simulink model "RobotSim"  (R2024b)
settings: Solver=ode45  StartTime=0.0  StopTime=100  MaxStep=0.1  RelTol=1e-3  EnableMultiTasking=on
InitFcn:
  | % LRS TU KL %
  | % By Alen Turnwald %
  | % 09.01.2017 %
  | clc
  | close
  | 
  | %% g_q
  | g_q = [1;0];
  | 
  | 
  | if ~exist('mp','var')||~exist('mc','var')||~exist('L','var')||~exist('g','var')||~exist('d1','var')||~exist('d2','var')
  | % Model Paramter
  |     warning(['(Some) Model Parameter are not defined!' ,10, '****  Setting the predefined parameter  ****'])
  |     N = 2;
  |     mc = 1.5;
  |     mp = 0.5;
  |     g = 9.82;
  |     L = 1;
  | % Damping factors
  |     d1 = 1e-2;
  |     d2 = 1e-2;
  | end
  | 
  | if ~exist('x_0','var')
  | % Initial state
  |     warning(['(Initial state "x_0" not defined or wrongly named!' ,10, '****  Setting x_0 = [0.1; 10 deg; 0; 0]  ****'])
  |     x_0 = zeros(4,1);
  |     x_0(1) = 0.1;
  |     x_0(2) = 10*pi/180;
  | end
  | 
  | if ~exist('K_lqr','var')||~exist('Kd_lqr','var')
  |     warning(['(No controller found!' ,10, '****   Applying a predefined controller  ****'])
  |     K_lqr = [-14.1421  171.8846  -25.2787   54.7535];
  | end
StopFcn:
  | %% load data
  | 
  | load output
  | 
  | %% Read data
  | q1 = out.Data(:,1);
  | q2 = out.Data(:,2)*180/pi;
  | x_ref = out.Data(:,5);
  | t = out.Time;
  | 
  | 
  | %% Plot
  | % close all
  | figure(2)
  | clf
  | h(1) = subplot(2,1,1);
  | plot(t,q1,'b','LineWidth',2); grid on
  | 
  | hold on
  | plot(t,x_ref,'r--')
  | hold off
  | ylabel('q_1 [m]')
  | legend('q_1','q_1 ref')
  | 
  | h(2) = subplot(2,1,2);
  | plot(t,q2,'b','LineWidth',2); grid on
  | hold on
  | plot(t,zeros(1,length(t)),'r--')
  | hold off
  | ylabel('q_2 [°]')
  | legend('q_2','q_2 ref')
  | 
  | xlabel('t [s]')
  | 
  | linkaxes(h,'x')
values from neighbouring files (symbols this model uses):
  l = 0.08    [robot.m]    (also in robot_cascade.m; robot_linear.m)
  m = 0.33    [robot.m]    (also in robot_cascade.m; robot_linear.m; robot_lqr.m)
  M = 1.180    (= 1.18)    [robot.m]    (also in robot_cascade.m; robot_linear.m; robot_lqr.m)
settings Model: Creator=Turnwald  LastModifiedBy=cosr3
settings SolverCC: AlgebraicLoopSolver=TrustRegion
settings DataIOCC: SaveFormat=Array  ReturnWorkspaceOutputs=off
settings OptimizationCC: OptimizeBlockIOStorage=off  BufferReuse=off  GlobalBufferReuse=off  ExpressionFolding=off  LocalBlockOutputs=off  LifeSpan=inf
settings DebuggingCC: SolverPrmCheckMsg=warning  UnconnectedInputMsg=warning  UnconnectedOutputMsg=warning  UnconnectedLineMsg=warning  AllowSymbolicDim=off  SFUnexpectedBacktrackingDiag=warning  SFNoUnconditionalDefaultTransitionDiag=warning  SFExecutionAtInitializationDiag=none  ArithmeticOperatorsInVariantConditions=warning
settings HardwareCC: ProdBitPerPointer=32  ProdBitPerSizeT=32  ProdBitPerPtrDiffT=32  ProdLargestAtomicFloat=None  ProdIntDivRoundTo=Undefined  ProdEndianess=Unspecified  ProdWordSize=32  ProdHWDeviceType=32-bit Generic
settings ModelReferenceCC: EnableRefExpFcnMdlSchedulingChecks=on  PropagateSignalLabelsOutOfModel=off
settings SFSimCC: SimUseLocalCustomCode=off  CustomCodeUndefinedFunction=UseInterfaceOnly
settings RTWCC: RTWUseLocalCustomCode=off  GPUComputeCapability=3.5
settings CodeAppCC: StateflowObjectComments=on
settings GRTTargetCC: TargetLangStandard=C89/C90 (ANSI)
settings ConfigComp: CovMetricSettings=dw  CovSaveCumulativeToWorkspaceVar=on  CovSaveSingleToWorkspaceVar=on  CovExternalEMLEnable=off

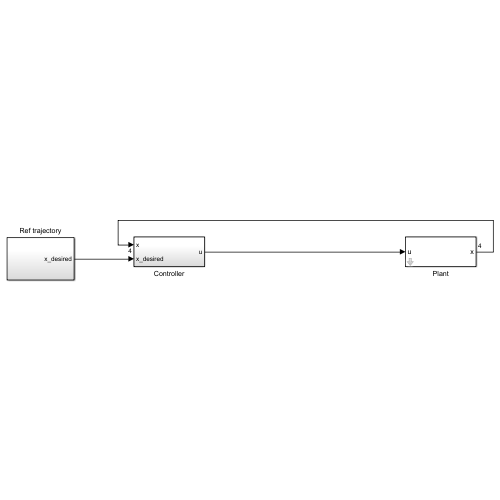
[thumbnail: Simulink's stored preview of the top-level diagram]
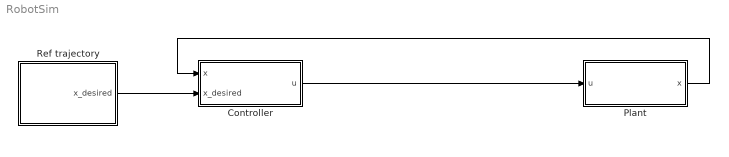
== system RobotSim ==
  Controller : Subsystem
  Plant : Subsystem  mask{mp=m, mc=M, L=l, g=g, g_q=g_q, d1=d1, d2=d2, x_0=x_0}
      mask help:
      | ---------------------------
      | TU Kaiserslautern, LRS
      | Ali Turnwald
      | Last Edit: 19.11.2015
      | ---------------------------
      |
      |
      | A non-linear model for the cart-pendulum system for simulation and animation
      |
      | mc = Mass of the cart
      | mp = Mass of the pendulum
      | g =  Earth gravity
      | L =  Length of the pendulum
      | d1 = Damping of the cart displacement
      | d2 = Damping in the joint
      | x_0 = The vector af initail state [4x1]
      mask DialogControl Text Prompt: Cart-Pendulum System
      mask Display:
      | port_label('output', 1, 'x')
      | port_label('input', 1, 'u')
  Ref trajectory : Subsystem
  wires:
  Ref trajectory/1(x_desired) -> Controller/2(x_desired)
  Plant/1(x) -> Controller/1(x)
  Controller/1(u) -> Plant/1(u)

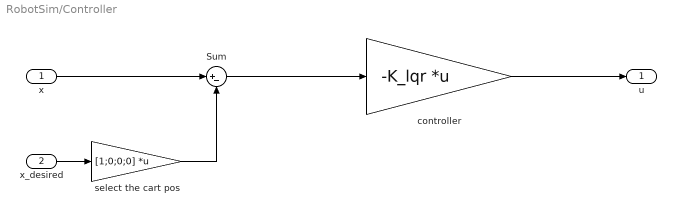
== system RobotSim/Controller ==
  x : Inport
  x_desired : Inport  Port=2
  Sum : Sum  Inputs=|+-
  controller : Gain  Gain=-K_lqr  Multiplication=Matrix(K*u)
  select the cart pos : Gain  Gain=[1;0;0;0]  Multiplication=Matrix(K*u)
  u : Outport  VectorParamsAs1DForOutWhenUnconnected=off
  wires:
  controller/1 -> u/1
  x_desired/1 -> select the cart pos/1
  x/1 -> Sum/1
  Sum/1 -> controller/1
  select the cart pos/1 -> Sum/2

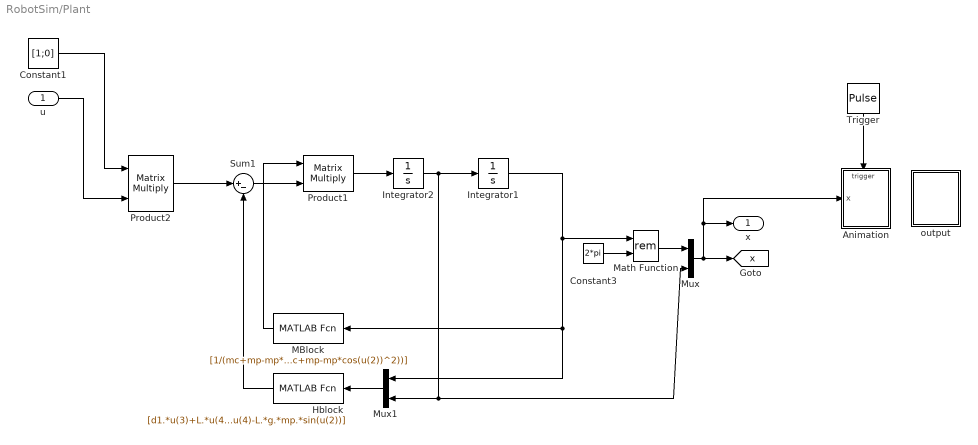
== system RobotSim/Plant ==
  u : Inport
  Animation : Subsystem
  Constant1 : Constant  Value=[1;0]
  Constant3 : Constant  Value=2*pi
  Hblock : MATLABFcn  MATLABFcn=[d1.*u(3)+L.*u(4).^2.*mp.*sin(u(2));d2.*u(4)-L.*g.*mp.*sin(u(2))]
  Integrator1 : Integrator  InitialCondition=x_0(1:2)
  Integrator2 : Integrator  InitialCondition=x_0(3:4)
  MBlock : MATLABFcn  MATLABFcn=[1/(mc+mp-mp*cos(u(2))^2),cos(u(2))/(L*(mc+mp-mp*cos(u(2))^2)); cos(u(2))/(L*(mc+mp-mp*cos(u(2))^2)), (mc+mp)/(L^2*mp*(mc+mp-mp*cos(u(2))^2))]  Output1D=off
  Math Function : Math  Operator=rem  SignedPower=on
  Mux : Mux  Inputs=2
  Mux1 : Mux  Inputs=2
  Product1 : Product  Multiplication=Matrix(*)
  Product2 : Product  Multiplication=Matrix(*)
  Sum1 : Sum  Inputs=|+-
  Trigger : DiscretePulseGenerator  PulseType=Time based  Period=0.1  PulseWidth=50
  output : Subsystem
  x : Outport  VectorParamsAs1DForOutWhenUnconnected=off
  tag scope: x=global
  wires:
  Integrator2/1 -> Mux1/2, Mux/2, Integrator1/1
  Product1/1 -> Integrator2/1
  Integrator1/1 -> Mux1/1, MBlock/1, Math Function/1
  MBlock/1 -> Product1/1
  Sum1/1 -> Product1/2
  Hblock/1 -> Sum1/2
  Constant1/1 -> Product2/1
  u/1 -> Product2/2
  Mux/1 -> [x], Animation/1(x), x/1
  Math Function/1 -> Mux/1
  Constant3/1 -> Math Function/2
  Product2/1 -> Sum1/1
  Trigger/1 -> Animation/Trigger
  Mux1/1 -> Hblock/1

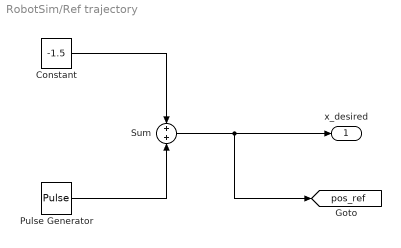
== system RobotSim/Ref trajectory ==
  Constant : Constant  Value=-1.5
  Pulse Generator : DiscretePulseGenerator  PulseType=Time based  Amplitude=3  Period=20  PulseWidth=50
  Sum : Sum
  x_desired : Outport  VectorParamsAs1DForOutWhenUnconnected=off
  tag scope: pos_ref=global
  wires:
  Sum/1 -> [pos_ref], x_desired/1
  Pulse Generator/1 -> Sum/2
  Constant/1 -> Sum/1

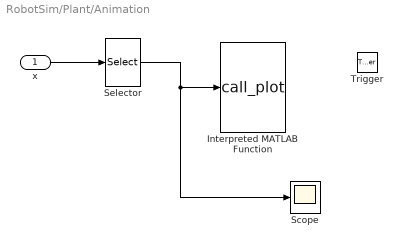
== system RobotSim/Plant/Animation ==
  x : Inport
  Trigger : TriggerPort  VariantControl=(inherit)  PortDimensions=1
  Interpreted MATLAB Function : MATLABFcn  MATLABFcn=call_plot  OutputDimensions=0
  Scope : Scope
  Selector : Selector  InputPortWidth=4  IndexOptions=Index vector (dialog)  Indices=[1:2]  OutputSizes=1
  wires:
  x/1 -> Selector/1
  Selector/1 -> Scope/1, Interpreted MATLAB Function/1

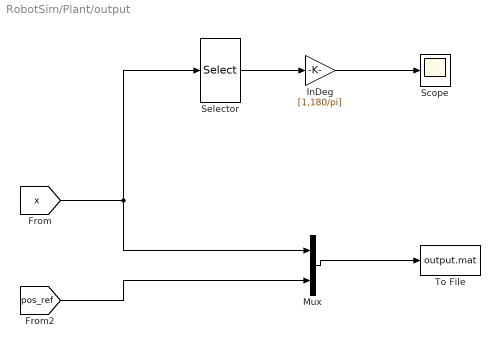
== system RobotSim/Plant/output ==
  InDeg : Gain  Gain=[1,180/pi]
  Mux : Mux  Inputs=2
  Scope : Scope
  Selector : Selector  InputPortWidth=4  IndexOptions=Index vector (dialog)  Indices=[1:2]  OutputSizes=1
  To File : ToFile  Filename=output.mat  MatrixName=out  SaveFormat=Timeseries
  wires:
  [x] -> Mux/1, Selector/1
  InDeg/1 -> Scope/1
  Selector/1 -> InDeg/1
  Mux/1 -> To File/1
  [pos_ref] -> Mux/2
